simulink model "model"  (R2020b)
settings: Solver=VariableStepAuto  StartTime=0.0  StopTime=10.0  MaxStep=0.001  RelTol=1e-3
settings Model: Creator=SAGAR  LastModifiedBy=SAGAR

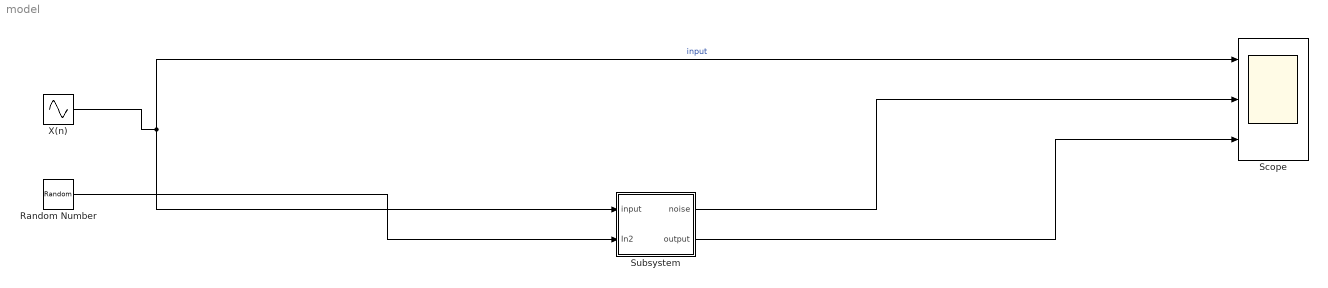
== system model ==
  Random Number : RandomNumber  SampleTime=0.1
  Scope : Scope  NumInputPorts=3
  Subsystem : Subsystem  TreatAsAtomicUnit=on
  X(n) : Sin  SampleTime=0.1
  wires:
  X(n)/1 -> Subsystem/1(input), Scope/1  "input"
  Random Number/1 -> Subsystem/2(In2)
  Subsystem/1(noise) -> Scope/2
  Subsystem/2(output) -> Scope/3

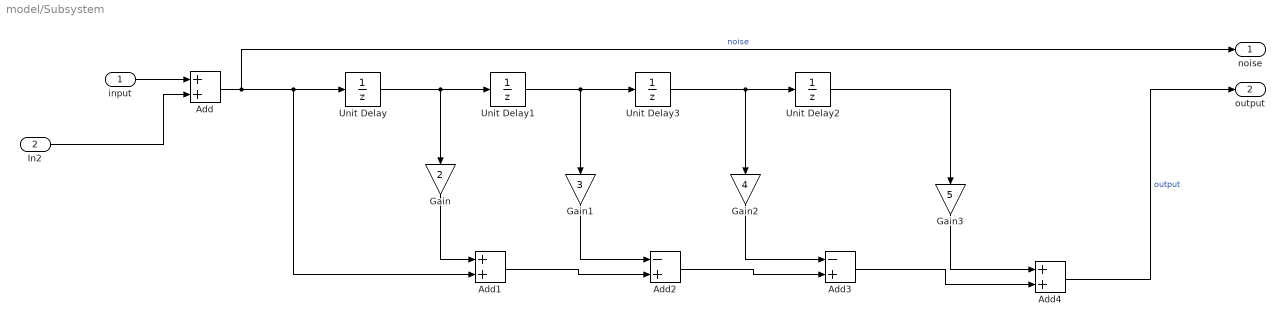
== system model/Subsystem ==
  input : Inport
  In2 : Inport  Port=2
  Add : Sum
  Add1 : Sum
  Add2 : Sum  Inputs=-+
  Add3 : Sum  Inputs=-+
  Add4 : Sum
  Gain : Gain  Gain=2
  Gain1 : Gain  Gain=3
  Gain2 : Gain  Gain=4
  Gain3 : Gain  Gain=5
  Unit Delay{,1..3} (4 alike) : UnitDelay  SampleTime=-1  HasFrameUpgradeWarning=on
  noise : Outport
  output : Outport  Port=2
  wires:
  Unit Delay2/1 -> Gain3/1
  Gain2/1 -> Add3/1
  Add2/1 -> Add3/2
  Unit Delay1/1 -> Gain1/1, Unit Delay3/1
  Unit Delay3/1 -> Gain2/1, Unit Delay2/1
  Add3/1 -> Add4/2
  Add/1 -> noise/1, Add1/2, Unit Delay/1  "noise"
  Gain3/1 -> Add4/1
  Unit Delay/1 -> Unit Delay1/1, Gain/1
  In2/1 -> Add/2
  Gain/1 -> Add1/1
  Add1/1 -> Add2/2
  Gain1/1 -> Add2/1
  input/1 -> Add/1
  Add4/1 -> output/1  "output"
